simulink model "Vehicle_Control_CodeGen"  (R2024a)
settings: Solver=FixedStepAuto  StartTime=0.0  StopTime=10  RelTol=1e-3  EnableMultiTasking=on
undefined symbols (not defined in the file or in its folder): CAN, DiscIntNeverNeededParam, FD, Ion, Lithium
libraries: stmutilitieslib x28, simulink x21, stm32blockslib x10, canfdmsglib x6, dspstat3 x6, slpidlib x3, spsBatteryLib x2, spsControlledCurrentSourceLib x2, spsVoltageMeasurementLib x2, spspowerguiLib x2, stm32h7xxblockslib x2
(part 2 of 3)

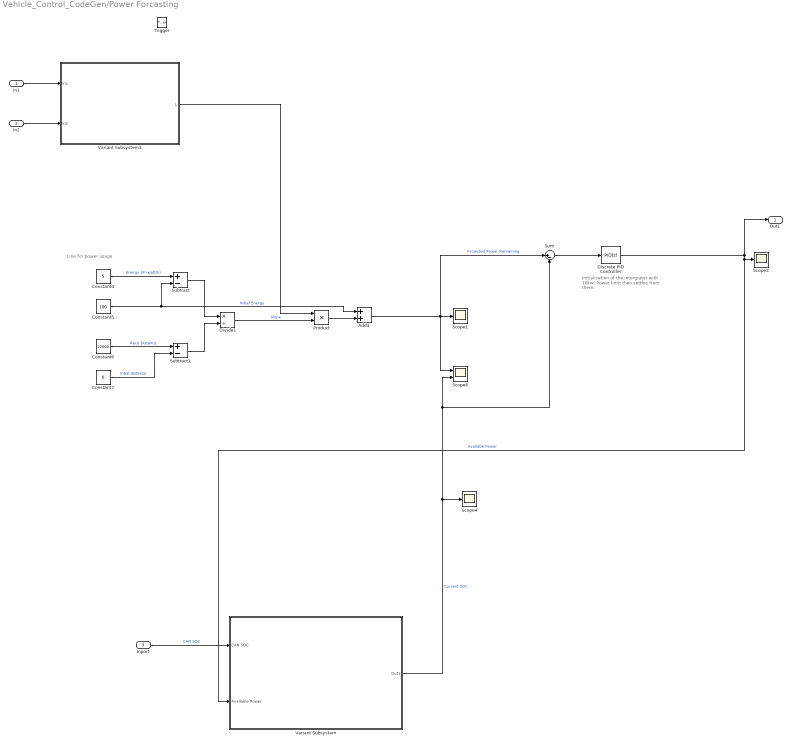
== system Vehicle_Control_CodeGen/Power Forcasting ==
  note: Line for power usage
  note: Initialisation of the intergrater with 10kw. Power limit then settles from there.
  In1 : Inport
  In2 : Inport  Port=2
  Inport : Inport  Port=3
  Trigger : TriggerPort  TriggerType=function-call  VariantControl=(inherit)
  Add3 : Sum
  Constant4 : Constant  Value=5
  Constant5 : Constant  Value=100
  Constant6 : Constant  Value=22000
  Constant7 : Constant  Value=0
  Discrete PID Controller : slpidlib/PID Controller  Controller=PID  Form=Parallel  TimeDomain=Discrete-time  UseExternalTs=off  SampleTime=-1  IntegratorMethod=Forward Euler  FilterMethod=Forward Euler  ControllerParametersSource=internal  P=-420  I=0.042  UseKiTs=off  D=21000  UseExternalDerivativeSource=off  N=0.01  UseFilter=on  TunerSelectOption=Transfer Function Based (PID Tuner App)  InitialConditionSource=internal  InitialConditionForIntegrator=10000  InitialConditionForFilter=0  DifferentiatorICPrevScaledInput=0  ExternalReset=none  TrackingMode=off  Kt=1  LimitOutput=off  SatLimitsSource=internal  UpperSaturationLimit=inf  LowerSaturationLimit=-inf  LinearizeAsGain=off  AntiWindupMode=none  Kb=1  LimitIntegrator=off  UpperIntegratorSaturationLimit=inf  LowerIntegratorSaturationLimit=-inf  POutMin=[]  POutMax=[]  IOutMin=[]  IOutMax=[]  DOutMin=[]  DOutMax=[]  NOutMin=[]  NOutMax=[]  SumOutMin=[]  SumOutMax=[]  SaturationOutMin=[]  SaturationOutMax=[]  PParamMin=[]  PParamMax=[]  IParamMin=[]  IParamMax=[]  DParamMin=[]  DParamMax=[]  NParamMin=[]  NParamMax=[]  KbParamMin=[]  KbParamMax=[]  KtParamMin=[]  KtParamMax=[]  KbOutMin=[]  KbOutMax=[]  KtOutMin=[]  KtOutMax=[]  IntegratorOutMin=[]  IntegratorOutMax=[]  FilterOutMin=[]  FilterOutMax=[]  SumI1OutMin=[]  SumI1OutMax=[]  SumI2OutMin=[]  SumI2OutMax=[]  SumI3OutMin=[]  SumI3OutMax=[]  SumI4OutMin=[]  SumI4OutMax=[]  SumDOutMin=[]  SumDOutMax=[]  DifferentiatorOutMin=[]  DifferentiatorOutMax=[]  FilterDiffOutCoefMin=[]  FilterDiffOutCoefMax=[]  ReciprocalOutMin=[]  ReciprocalOutMax=[]  SumDenOutMin=[]  SumDenOutMax=[]  SumNumOutMin=[]  SumNumOutMax=[]  DivideOutMin=[]  DivideOutMax=[]  UdiffTsProdOutMin=[]  UdiffTsProdOutMax=[]  NTsProdOutMin=[]  NTsProdOutMax=[]  UintegralTsProdOutMin=[]  UintegralTsProdOutMax=[]  UngainTsProdOutMin=[]  UngainTsProdOutMax=[]  ClampingZeroOutDataTypeStr=Inherit: Inherit via back propagation  ClampingZeroOutMin=[]  ClampingZeroOutMax=[]  FilterDenConstantOutDataTypeStr=Inherit: Inherit via back propagation  FilterDenConstantOutMin=[]  FilterDenConstantOutMax=[]  PCopyOutDataTypeStr=Inherit: Inherit via back propagation  PCopyOutMin=[]  PCopyOutMax=[]  NCopyOutDataTypeStr=Inherit: Inherit via back propagation  NCopyOutMin=[]  NCopyOutMax=[]  IntegratorContinuousStateAttributes=''  IntegratorStateMustResolveToSignalObject=off  IntegratorRTWStateStorageClass=Auto  FilterContinuousStateAttributes=''  FilterStateMustResolveToSignalObject=off  FilterRTWStateStorageClass=Auto  ParallelPVariant=InternalParameters  IdealPVariant=Disabled  IVariant=InternalParameters  DVariant=InternalParameters  IntegratorVariant=Discrete  SatVariant=Disabled  AWVariant=Passthrough  PCopyVariant=Disabled  TRVariant=Disabled  FdbkBlocksVariant=Forward  IdealPFdbkVariant=Disabled  SatFdbkVariant=Disabled  DerivativeFilterVariant=ForwardEulerFilter  NVariant=InternalParameters  NCopyVariant=Disabled  FilterICVariant=InternalICsFilter  IntegratorICVariant=InternalICs  ExternalResetVariant=Disabled  TRSumVariant=Passthrough  SumFdbkVariant=Disabled  SumVariant=Sum_PID  TsampFilterVariant=InternalTs  TsampNgainVariant=Passthrough  TsampIntegralVariant=Disabled_SignalSpec  ExternalSaturationOutDataTypeStr=Inherit: Same as second input  DerivativeSourceVariant=ErrorSignal
      settings: LibrarySourceBlock=simulink/Discrete/Discrete PID Controller
  Divide1 : Product  Inputs=*/
  Product : Product
  Scope1 : Scope
  Scope3 : Scope
  Scope4 : Scope
  Scope6 : Scope  NumInputPorts=2
  Subtract : Sum  Inputs=+-
  Subtract1 : Sum  Inputs=+-
  Sum : Sum  Inputs=|+-
  Variant Subsystem : Subsystem  Variant=on  VariantControlMode=sim codegen switching
  Variant Subsystem1 : Subsystem  Variant=on  VariantControlMode=sim codegen switching
  Out1 : Outport
  wires:
  In1/1 -> Variant Subsystem1/1(In1)
  In2/1 -> Variant Subsystem1/2(In2)
  Variant Subsystem/1(Out1) -> Scope4/1, Sum/2, Scope6/2  "Current SOC"
  Variant Subsystem1/1(1) -> Product/1
  Constant7/1 -> Subtract1/2  "Intial distance"
  Sum/1 -> Discrete PID Controller/1
  Divide1/1 -> Product/2  "Slope"
  Subtract1/1 -> Divide1/2
  Product/1 -> Add3/2
  Add3/1 -> Scope6/1, Sum/1, Scope1/1  "Projected Power Remaining"
  Constant4/1 -> Subtract/1  "Energy SF (watt/h)"
  Discrete PID Controller/1 -> Variant Subsystem/2(Available Power), Scope3/1, Out1/1  "Availabe Power"
  Constant5/1 -> Add3/1, Subtract/2  "Initial Energy"
  Subtract/1 -> Divide1/1
  Constant6/1 -> Subtract1/1  "Race Distance"
  Inport/1 -> Variant Subsystem/1(CAN SOC)  "CAN SOC"

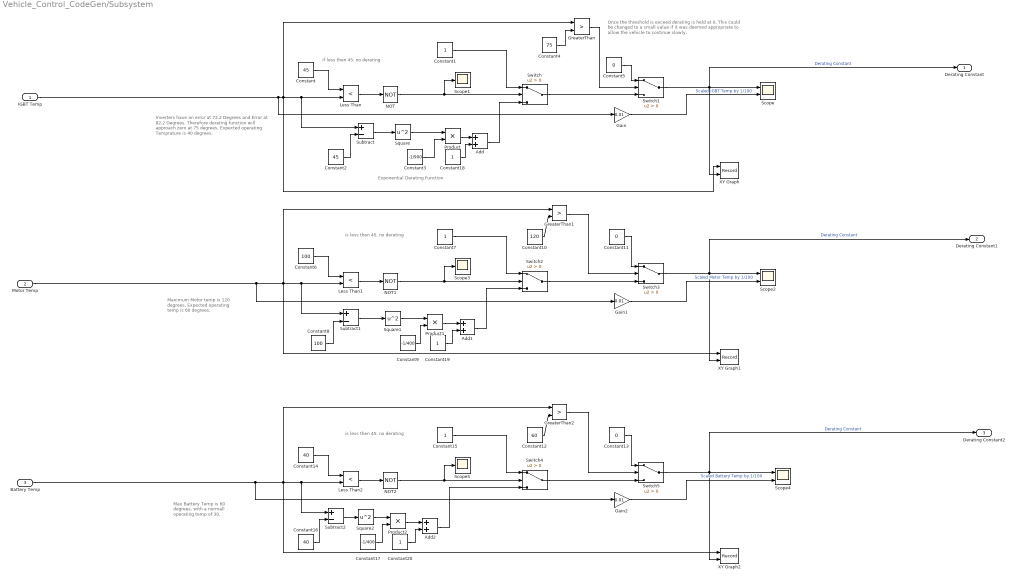
== system Vehicle_Control_CodeGen/Subsystem ==
  note: Once the threshold is exceed derating is held at 0, This could be changed to a small value if it was deemed appropriate to allow the vehicle to continue slowly.
  note: Exponential Derating Function
  note: if less then 45, no derating
  note: Max Battery Temp is 60 degrees, with a normall operating temp of 30.
  note: Maximum Motor temp is 120 degrees. Expected operating temp is 60 degrees.
  note: Inverters have an error at 72.2 Degrees and Error at 82.2 Degrees. Therefore derating function will approach zero at 75 degrees. Expected operating Temprature is 40 degrees.
  note: is less then 45, no derating
  note: is less then 45, no derating
  IGBT Temp : Inport
  Motor Temp : Inport  Port=2
  Battery Temp : Inport  Port=3
  Add : Sum
  Add1 : Sum
  Add2 : Sum
  Constant : Constant  Value=45
  Constant{1,7,15,18..20} (6 alike) : Constant
  Constant10 : Constant  Value=120
  Constant11 : Constant  Value=0
  Constant12 : Constant  Value=60
  Constant13 : Constant  Value=0
  Constant14 : Constant  Value=40
  Constant16 : Constant  Value=40
  Constant17 : Constant  Value=-1/400
  Constant2 : Constant  Value=45
  Constant3 : Constant  Value=-1/900
  Constant4 : Constant  Value=75
  Constant5 : Constant  Value=0
  Constant6 : Constant  Value=100
  Constant8 : Constant  Value=100
  Constant9 : Constant  Value=-1/400
  Gain : Gain  Gain=0.01
  Gain1 : Gain  Gain=0.01
  Gain2 : Gain  Gain=0.01
  GreaterThan : RelationalOperator  Operator=>  OutDataTypeStr=boolean  RndMeth=Simplest  InputSameDT=off
  GreaterThan1 : RelationalOperator  Operator=>  OutDataTypeStr=boolean  RndMeth=Simplest  InputSameDT=off
  GreaterThan2 : RelationalOperator  Operator=>  OutDataTypeStr=boolean  RndMeth=Simplest  InputSameDT=off
  Less Than : RelationalOperator  Operator=<  OutDataTypeStr=boolean  RndMeth=Simplest  InputSameDT=off
  Less Than1 : RelationalOperator  Operator=<  OutDataTypeStr=boolean  RndMeth=Simplest  InputSameDT=off
  Less Than2 : RelationalOperator  Operator=<  OutDataTypeStr=boolean  RndMeth=Simplest  InputSameDT=off
  NOT : Logic  Operator=NOT  IconShape=distinctive  AllPortsSameDT=off  OutDataTypeStr=boolean
  NOT1 : Logic  Operator=NOT  IconShape=distinctive  AllPortsSameDT=off  OutDataTypeStr=boolean
  NOT2 : Logic  Operator=NOT  IconShape=distinctive  AllPortsSameDT=off  OutDataTypeStr=boolean
  Product : Product
  Product1 : Product
  Product2 : Product
  Scope : Scope  NumInputPorts=2
  Scope1 : Scope
  Scope2 : Scope  NumInputPorts=2
  Scope3 : Scope
  Scope4 : Scope  NumInputPorts=2
  Scope5 : Scope
  Square : Math  Operator=square
  Square1 : Math  Operator=square
  Square2 : Math  Operator=square
  Subtract : Sum  Inputs=+-
  Subtract1 : Sum  Inputs=+-
  Subtract2 : Sum  Inputs=+-
  Switch{,1..5} (6 alike) : Switch  Criteria=u2 > Threshold  SaturateOnIntegerOverflow=off  InputSameDT=off
  XY Graph : Record  FileSettingsInternal="{\"entries\":[{\"content\":{\"excelSettings\":{\"content\":{},\"type\":\"Streamout.ExcelSettings\"}},\"type\":\"Streamout.FileSettingStorage\",\"uuid\":\"\"}],\"packageUris\":[\"http:\\/\\/schema.mathworks.com\\/mf0\\/streamout_blocks\\/R2020a\"],\"version\":\"1.0\"}"  Layout=[1 1]  SignalsInternal="{\"entries\":[{\"content\":{\"signals\":[{\"content\":{\"blockPath\":[],\"dimensions\":[1],\"domain\":\"\",\"lineColor\":\"#a2142f\",\"plots\":[ 1 ],\"port\":1,\"signalID\":1,\"signalName\":\"IGBT Temp\"},\"type\":\"RecordBlkView.Signal\",\"uuid\":\"\"},{\"content\":{\"blockPath\":[],\"dimensions\":[1],\"domain\":\"\",\"lineColor\":\"#139fff\",\"plots\":[ 1 ],\"port\":2,\"signalID\":2,\"signalName\":\"Derating Constant\"},\"type\":\"RecordBlkView.Signal\",\"uuid\":\"\"}]},\"type\":\"RecordBlkView.InputSignals\",\"uuid\":\"\"}],\"packageUris\":[\"http:\\/\\/schema.mathworks.com\\/mf0\\/streamout_blocks\\/R2020a\"],\"version\":\"1.0\"}"  VisualizationBindings="{\"xyplotplugin\":{\"info\":[{\"series\":[{\"bindingParametersList\":[{\"parameter\":\"X-Axis\",\"signalID\":1,\"signalName\":\"IGBT Temp\"},{\"parameter\":\"Y-Axis\",\"signalID\":2,\"signalName\":\"Derating Constant\"}],\"seriesID\":0}],\"subplotID\":1}]}}"  CompatibilityTag=XY
  XY Graph1 : Record  FileSettingsInternal="{\"entries\":[{\"content\":{\"excelSettings\":{\"content\":{},\"type\":\"Streamout.ExcelSettings\"}},\"type\":\"Streamout.FileSettingStorage\",\"uuid\":\"\"}],\"packageUris\":[\"http:\\/\\/schema.mathworks.com\\/mf0\\/streamout_blocks\\/R2020a\"],\"version\":\"1.0\"}"  Layout=[1 1]  SignalsInternal="{\"entries\":[{\"content\":{\"signals\":[{\"content\":{\"blockPath\":[],\"dimensions\":[1],\"domain\":\"\",\"lineColor\":\"#a2142f\",\"plots\":[ 1 ],\"port\":1,\"signalID\":1,\"signalName\":\"Motor Temp\"},\"type\":\"RecordBlkView.Signal\",\"uuid\":\"\"},{\"content\":{\"blockPath\":[],\"dimensions\":[1],\"domain\":\"\",\"lineColor\":\"#139fff\",\"plots\":[ 1 ],\"port\":2,\"signalID\":2,\"signalName\":\"Derating Constant\"},\"type\":\"RecordBlkView.Signal\",\"uuid\":\"\"}]},\"type\":\"RecordBlkView.InputSignals\",\"uuid\":\"\"}],\"packageUris\":[\"http:\\/\\/schema.mathworks.com\\/mf0\\/streamout_blocks\\/R2020a\"],\"version\":\"1.0\"}"  VisualizationBindings="{\"xyplotplugin\":{\"info\":[{\"series\":[{\"bindingParametersList\":[{\"parameter\":\"X-Axis\",\"signalID\":1,\"signalName\":\"Motor Temp\"},{\"parameter\":\"Y-Axis\",\"signalID\":2,\"signalName\":\"Derating Constant\"}],\"seriesID\":0}],\"subplotID\":1}]}}"  CompatibilityTag=XY
  XY Graph2 : Record  FileSettingsInternal="{\"entries\":[{\"content\":{\"excelSettings\":{\"content\":{},\"type\":\"Streamout.ExcelSettings\"}},\"type\":\"Streamout.FileSettingStorage\",\"uuid\":\"\"}],\"packageUris\":[\"http:\\/\\/schema.mathworks.com\\/mf0\\/streamout_blocks\\/R2020a\"],\"version\":\"1.0\"}"  Layout=[1 1]  SignalsInternal="{\"entries\":[{\"content\":{\"signals\":[{\"content\":{\"blockPath\":[],\"dimensions\":[1],\"domain\":\"\",\"lineColor\":\"#a2142f\",\"plots\":[ 1 ],\"port\":1,\"signalID\":1,\"signalName\":\"Battery Temp\"},\"type\":\"RecordBlkView.Signal\",\"uuid\":\"\"},{\"content\":{\"blockPath\":[],\"dimensions\":[1],\"domain\":\"\",\"lineColor\":\"#139fff\",\"plots\":[ 1 ],\"port\":2,\"signalID\":2,\"signalName\":\"Derating Constant\"},\"type\":\"RecordBlkView.Signal\",\"uuid\":\"\"}]},\"type\":\"RecordBlkView.InputSignals\",\"uuid\":\"\"}],\"packageUris\":[\"http:\\/\\/schema.mathworks.com\\/mf0\\/streamout_blocks\\/R2020a\"],\"version\":\"1.0\"}"  VisualizationBindings="{\"xyplotplugin\":{\"info\":[{\"series\":[{\"bindingParametersList\":[{\"parameter\":\"X-Axis\",\"signalID\":1,\"signalName\":\"Battery Temp\"},{\"parameter\":\"Y-Axis\",\"signalID\":2,\"signalName\":\"Derating Constant\"}],\"seriesID\":0}],\"subplotID\":1}]}}"  CompatibilityTag=XY
  Derating Constant : Outport
  Derating Constant1 : Outport  Port=2
  Derating Constant2 : Outport  Port=3
  wires:
  Add/1 -> Switch/3
  Less Than2/1 -> NOT2/1
  Motor Temp/1 -> XY Graph1/1, GreaterThan1/1, Subtract1/1, Less Than1/2, Gain1/1
  NOT2/1 -> Scope5/1, Switch4/2
  Constant7/1 -> Switch2/1
  Switch1/1 -> Derating Constant/1, Scope/1, XY Graph/2  "Derating Constant"
  Gain1/1 -> Scope2/2  "Scaled Motor Temp by 1/100"
  NOT1/1 -> Scope3/1, Switch2/2
  GreaterThan/1 -> Switch1/2
  Constant18/1 -> Add/2
  Constant16/1 -> Subtract2/2
  Subtract1/1 -> Square1/1
  Constant1/1 -> Switch/1
  Battery Temp/1 -> XY Graph2/1, GreaterThan2/1, Subtract2/1, Less Than2/2, Gain2/1
  Subtract2/1 -> Square2/1
  Constant5/1 -> Switch1/1
  Switch/1 -> Switch1/3
  Less Than/1 -> NOT/1
  Product1/1 -> Add1/1
  Constant2/1 -> Subtract/2
  Constant6/1 -> Less Than1/1
  Subtract/1 -> Square/1
  Gain2/1 -> Scope4/2  "Scaled Battery Temp by 1/100"
  Add1/1 -> Switch2/3
  Add2/1 -> Switch4/3
  Constant19/1 -> Add1/2
  Constant8/1 -> Subtract1/2
  Square/1 -> Product/1
  Constant9/1 -> Product1/2
  Constant4/1 -> GreaterThan/2
  IGBT Temp/1 -> Gain/1, XY Graph/1, GreaterThan/1, Subtract/1, Less Than/2
  Constant10/1 -> GreaterThan1/2
  Gain/1 -> Scope/2  "Scaled IGBT Temp by 1/100"
  Switch2/1 -> Switch3/3
  Switch3/1 -> Derating Constant1/1, Scope2/1, XY Graph1/2  "Derating Constant"
  Constant3/1 -> Product/2
  Constant14/1 -> Less Than2/1
  Constant20/1 -> Add2/2
  Switch4/1 -> Switch5/3
  Square1/1 -> Product1/1
  Less Than1/1 -> NOT1/1
  Constant11/1 -> Switch3/1
  Constant12/1 -> GreaterThan2/2
  Square2/1 -> Product2/1
  GreaterThan1/1 -> Switch3/2
  Switch5/1 -> Derating Constant2/1, Scope4/1, XY Graph2/2  "Derating Constant"
  Constant13/1 -> Switch5/1
  Product/1 -> Add/1
  Constant/1 -> Less Than/1
  Constant15/1 -> Switch4/1
  NOT/1 -> Scope1/1, Switch/2
  Product2/1 -> Add2/1
  Constant17/1 -> Product2/2
  GreaterThan2/1 -> Switch5/2

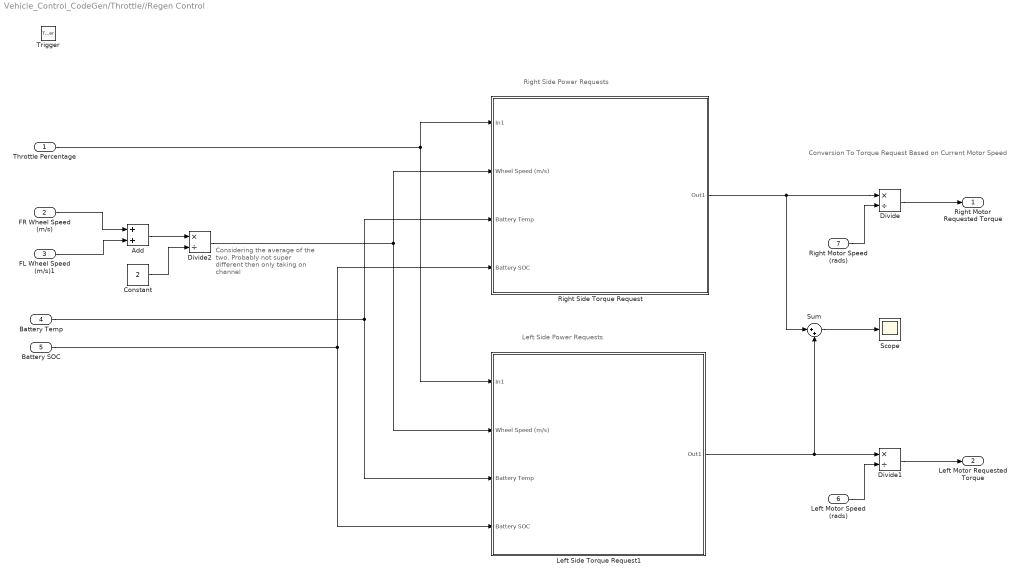
== system Vehicle_Control_CodeGen/Throttle//Regen Control ==
  note: Conversion To Torque Request Based on Current Motor Speed
  note: Right Side Power Requests
  note: Considering the average of the two. Probably not super different then only taking on channel
  note: Left Side Power Requests
  Throttle Percentage : Inport
  FR Wheel Speed (m/s) : Inport  Port=2
  FL Wheel Speed (m/s)1 : Inport  Port=3
  Battery Temp : Inport  Port=4
  Battery SOC : Inport  Port=5
  Left Motor Speed (rads) : Inport  Port=6
  Right Motor Speed (rads) : Inport  Port=7
  Trigger : TriggerPort  TriggerType=function-call  VariantControl=(inherit)
  Add : Sum
  Constant : Constant  Value=2
  Divide : Product  Inputs=*/
  Divide1 : Product  Inputs=*/
  Divide2 : Product  Inputs=*/
  Left Side Torque Request1 : Subsystem
  Right Side Torque Request : Subsystem
  Scope : Scope
  Sum : Sum  Inputs=|++
  Right Motor Requested Torque : Outport
  Left Motor Requested Torque : Outport  Port=2
  wires:
  Right Side Torque Request/1(Out1) -> Sum/1, Divide/1
  Divide/1 -> Right Motor Requested Torque/1
  Left Motor Speed (rads)/1 -> Divide1/2
  Sum/1 -> Scope/1
  Left Side Torque Request1/1(Out1) -> Divide1/1, Sum/2
  Divide1/1 -> Left Motor Requested Torque/1
  Throttle Percentage/1 -> Left Side Torque Request1/1(In1), Right Side Torque Request/1(In1)
  Right Motor Speed (rads)/1 -> Divide/2
  Divide2/1 -> Right Side Torque Request/2(Wheel Speed (m/s)), Left Side Torque Request1/2(Wheel Speed (m/s))
  Battery Temp/1 -> Right Side Torque Request/3(Battery Temp), Left Side Torque Request1/3(Battery Temp)
  Battery SOC/1 -> Right Side Torque Request/4(Battery SOC), Left Side Torque Request1/4(Battery SOC)
  FR Wheel Speed (m/s)/1 -> Add/1
  FL Wheel Speed (m/s)1/1 -> Add/2
  Add/1 -> Divide2/1
  Constant/1 -> Divide2/2

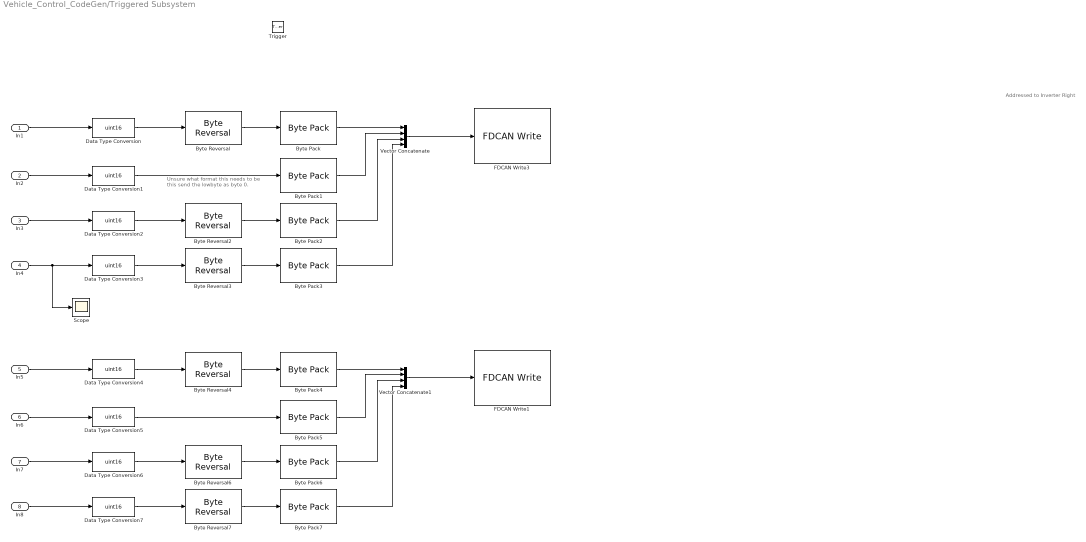
== system Vehicle_Control_CodeGen/Triggered Subsystem ==
  note: Unsure what format this needs to be this send the lowbyte as byte 0.
  note: Addressed to Inverter Right
  In1 : Inport
  In2 : Inport  Port=2
  In3 : Inport  Port=3
  In4 : Inport  Port=4
  In5 : Inport  Port=5
  In6 : Inport  Port=6
  In7 : Inport  Port=7
  In8 : Inport  Port=8
  Trigger : TriggerPort  TriggerType=function-call  VariantControl=(inherit)
  Byte Pack{,1..7} (8 alike) : stmutilitieslib/Byte Pack  datatypes={'uint16'}  byteAlign=1  blockPlatform=stm32f4discovery
  Byte Reversal{,2..4,6..7} (6 alike) : stmutilitieslib/Byte Reversal  numInp=1  blockPlatform=stm32f4discovery
  Data Type Conversion{,1..7} (8 alike) : DataTypeConversion  OutDataTypeStr=uint16  SaturateOnIntegerOverflow=off  RndMeth=Floor
  FDCAN Write1 : stm32blockslib/FDCAN Write  FDCANModule=FDCAN2  BlockMode=Transmit  OperationReadMode=Data  OperationWriteMode=Data  ReadSource=FIFO 0  BufferNumber=0  OutputTypeReadMode=Unpacked  DataFormatWriteMode=Raw data  CANFrameType=CAN  IdentifierTypeVia=Dialog  IdentifierType=Standard (11-bit identifier)  IdentifierVia=Dialog  Identifier=9  DataLengthVia=Dialog  DataLength=8  OutputIdType=off  IsBitRateSwitchingEnabled=off  TransmitRemoteFrame=off  OutputFrameType=off  OutputBRS=off  OutputRemoteFrame=off  OutputTxFifoLevel=off  OutputRxFifoLevel=off  OutputStatus=off  Timeout=1  SampleTime=-1
      settings: LibrarySourceBlock=stm32l5xxblockslib/FDCAN Write
  FDCAN Write3 : stm32blockslib/FDCAN Write  FDCANModule=FDCAN2  BlockMode=Transmit  OperationReadMode=Data  OperationWriteMode=Data  ReadSource=FIFO 0  BufferNumber=0  OutputTypeReadMode=Unpacked  DataFormatWriteMode=Raw data  CANFrameType=CAN  IdentifierTypeVia=Dialog  IdentifierType=Standard (11-bit identifier)  IdentifierVia=Dialog  Identifier=8  DataLengthVia=Dialog  DataLength=8  OutputIdType=off  IsBitRateSwitchingEnabled=off  TransmitRemoteFrame=off  OutputFrameType=off  OutputBRS=off  OutputRemoteFrame=off  OutputTxFifoLevel=off  OutputRxFifoLevel=off  OutputStatus=off  Timeout=1  SampleTime=-1
      settings: LibrarySourceBlock=stm32l5xxblockslib/FDCAN Write
  Scope : Scope
  Vector Concatenate : Concatenate  NumInputs=4
  Vector Concatenate1 : Concatenate  NumInputs=4
  wires:
  Byte Reversal/1 -> Byte Pack/1
  Byte Pack/1 -> Vector Concatenate/1
  Data Type Conversion/1 -> Byte Reversal/1
  In1/1 -> Data Type Conversion/1
  Byte Pack1/1 -> Vector Concatenate/2
  Byte Pack2/1 -> Vector Concatenate/3
  Byte Reversal2/1 -> Byte Pack2/1
  Data Type Conversion2/1 -> Byte Reversal2/1
  Byte Pack3/1 -> Vector Concatenate/4
  Byte Reversal3/1 -> Byte Pack3/1
  Data Type Conversion3/1 -> Byte Reversal3/1
  In3/1 -> Data Type Conversion2/1
  In4/1 -> Scope/1, Data Type Conversion3/1
  Vector Concatenate/1 -> FDCAN Write3/1
  Byte Pack6/1 -> Vector Concatenate1/3
  Byte Reversal7/1 -> Byte Pack7/1
  Vector Concatenate1/1 -> FDCAN Write1/1
  Byte Pack5/1 -> Vector Concatenate1/2
  Byte Pack7/1 -> Vector Concatenate1/4
  Byte Pack4/1 -> Vector Concatenate1/1
  Data Type Conversion7/1 -> Byte Reversal7/1
  Data Type Conversion4/1 -> Byte Reversal4/1
  Data Type Conversion5/1 -> Byte Pack5/1
  Byte Reversal6/1 -> Byte Pack6/1
  Data Type Conversion6/1 -> Byte Reversal6/1
  Byte Reversal4/1 -> Byte Pack4/1
  In8/1 -> Data Type Conversion7/1
  In7/1 -> Data Type Conversion6/1
  In6/1 -> Data Type Conversion5/1
  In5/1 -> Data Type Conversion4/1
  Data Type Conversion1/1 -> Byte Pack1/1
  In2/1 -> Data Type Conversion1/1

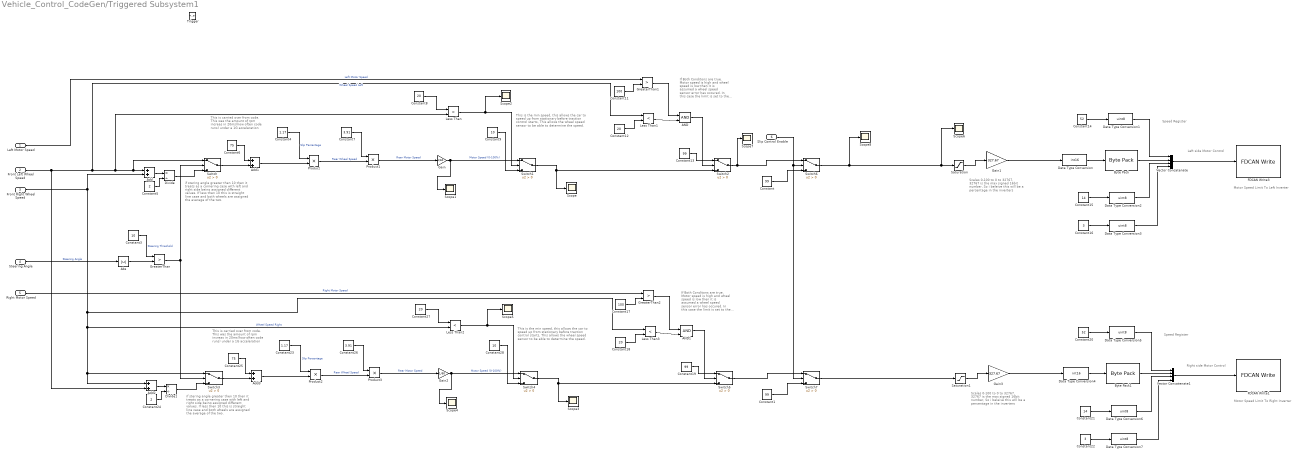
== system Vehicle_Control_CodeGen/Triggered Subsystem1 ==
  note: Scales 0-100 to 0 to 32767, 32767 is the max signed 16bit number, So i beleive this will be a percentage in the inverters
  note: Left side Motor Control
  note: If Both Conditons are true. Motor speed is high and wheel speed is low then it is assumed a wheel speed sensor error has occured. In this case the limit is set to the maximum.
  note: Speed Register
  note: Speed Register
  note: if stering angle greater then 10 then it treats as a cornering case with left and right side being assigned different values. If less then 10 this is straight line case and both wheels are assigned the average of the two.
  note: This is carried over from code. This was the amount of rpm increas in 20ms(how often code runs) under a 1G acceleration
  note: This is the min speed, this allows the car to speed up from stationary before traction control starts, This allows the wheel speed sensor to be able to determine the speed.
  note: if stering angle greater then 10 then it treats as a cornering case with left and right side being assigned different values. If less then 10 this is straight line case and both wheels are assigned the average of the two.
  note: This is the min speed, this allows the car to speed up from stationary before traction control starts, This allows the wheel speed sensor to be able to determine the speed.
  note: If Both Conditons are true. Motor speed is high and wheel speed is low then it is assumed a wheel speed sensor error has occured. In this case the limit is set to the maximum.
  note: Right side Motor Control
  note: Scales 0-100 to 0 to 32767, 32767 is the max signed 16bit number, So i beleive this will be a percentage in the inverters
  note: This is carried over from code. This was the amount of rpm increas in 20ms(how often code runs) under a 1G acceleration
  note: Motor Speed Limit To Right Inverter
  note: Motor Speed Limit To Left Inverter
  Left Motor Speed : Inport
  Front Left Wheel Speed : Inport  Port=2
  Front Right Wheel Speed : Inport  Port=3
  Steering Angle : Inport  Port=4
  Right Motor Speed : Inport  Port=5
  Slip Control Enable : Inport  Port=6
  Trigger : TriggerPort  TriggerType=function-call  VariantControl=(inherit)
  AND : Logic  IconShape=distinctive  AllPortsSameDT=off  OutDataTypeStr=boolean
  AND1 : Logic  IconShape=distinctive  AllPortsSameDT=off  OutDataTypeStr=boolean
  Abs : Abs  SaturateOnIntegerOverflow=off
  Add{,1..3} (4 alike) : Sum
  Byte Pack : stmutilitieslib/Byte Pack  datatypes={'int16'}  byteAlign=1  blockPlatform=stm32f4discovery
  Byte Pack1 : stmutilitieslib/Byte Pack  datatypes={'int16'}  byteAlign=1  blockPlatform=stm32f4discovery
  Constant{,1,13,19} (4 alike) : Constant  Value=99
  Constant11 : Constant  Value=100
  Constant{8,12,18,27} (4 alike) : Constant  Value=20
  Constant14 : Constant  Value=52
  Constant15 : Constant  Value=14
  Constant16 : Constant  Value=3
  Constant17 : Constant  Value=100
  Constant20 : Constant  Value=52
  Constant21 : Constant  Value=14
  Constant22 : Constant  Value=3
  Constant23 : Constant  Value=1.17
  Constant24 : Constant  Value=2
  Constant25 : Constant  Value=75
  Constant26 : Constant  Value=3.91
  Constant28 : Constant  Value=10
  Constant3 : Constant  Value=10
  Constant4 : Constant  Value=1.17
  Constant5 : Constant  Value=2
  Constant6 : Constant  Value=75
  Constant7 : Constant  Value=3.91
  Constant9 : Constant  Value=10
  Data Type Conversion : DataTypeConversion  OutDataTypeStr=int16  SaturateOnIntegerOverflow=off  RndMeth=Floor
  Data Type Conversion{1..3,5..7} (6 alike) : DataTypeConversion  OutDataTypeStr=uint8  SaturateOnIntegerOverflow=off  RndMeth=Floor
  Data Type Conversion4 : DataTypeConversion  OutDataTypeStr=int16  SaturateOnIntegerOverflow=off  RndMeth=Floor
  Divide : Product  Inputs=*/
  Divide1 : Product  Inputs=*/
  FDCAN Write1 : stm32blockslib/FDCAN Write  FDCANModule=FDCAN2  BlockMode=Transmit  OperationReadMode=Data  OperationWriteMode=Data  ReadSource=FIFO 0  BufferNumber=0  OutputTypeReadMode=Unpacked  DataFormatWriteMode=Raw data  CANFrameType=CAN  IdentifierTypeVia=Dialog  IdentifierType=Standard (11-bit identifier)  IdentifierVia=Dialog  Identifier=529  DataLengthVia=Dialog  DataLength=3  OutputIdType=off  IsBitRateSwitchingEnabled=off  TransmitRemoteFrame=off  OutputFrameType=off  OutputBRS=off  OutputRemoteFrame=off  OutputTxFifoLevel=off  OutputRxFifoLevel=off  OutputStatus=off  Timeout=1  SampleTime=-1
      settings: LibrarySourceBlock=stm32l5xxblockslib/FDCAN Write
  FDCAN Write3 : stm32blockslib/FDCAN Write  FDCANModule=FDCAN2  BlockMode=Transmit  OperationReadMode=Data  OperationWriteMode=Data  ReadSource=FIFO 0  BufferNumber=0  OutputTypeReadMode=Unpacked  DataFormatWriteMode=Raw data  CANFrameType=CAN  IdentifierTypeVia=Dialog  IdentifierType=Standard (11-bit identifier)  IdentifierVia=Dialog  Identifier=528  DataLengthVia=Dialog  DataLength=3  OutputIdType=off  IsBitRateSwitchingEnabled=off  TransmitRemoteFrame=off  OutputFrameType=off  OutputBRS=off  OutputRemoteFrame=off  OutputTxFifoLevel=off  OutputRxFifoLevel=off  OutputStatus=off  Timeout=1  SampleTime=-1
      settings: LibrarySourceBlock=stm32l5xxblockslib/FDCAN Write
  Gain : Gain  Gain=1/60
  Gain1 : Gain  Gain=327.67
  Gain2 : Gain  Gain=1/60
  Gain3 : Gain  Gain=327.67
  GreaterThan : RelationalOperator  Operator=>  OutDataTypeStr=boolean  RndMeth=Simplest  InputSameDT=off
  GreaterThan1 : RelationalOperator  Operator=>  OutDataTypeStr=boolean  RndMeth=Simplest  InputSameDT=off
  GreaterThan2 : RelationalOperator  Operator=>  OutDataTypeStr=boolean  RndMeth=Simplest  InputSameDT=off
  Less Than{,1..3} (4 alike) : RelationalOperator  Operator=<  OutDataTypeStr=boolean  RndMeth=Simplest  InputSameDT=off
  Product{,1..3} (4 alike) : Product
  Saturation : Saturate  UpperLimit=99  LowerLimit=0
  Saturation1 : Saturate  UpperLimit=99  LowerLimit=0
  Scope{,1..8} (9 alike) : Scope
  Switch{,1..7} (8 alike) : Switch  Criteria=u2 > Threshold  SaturateOnIntegerOverflow=off  InputSameDT=off
  Vector Concatenate : Concatenate  NumInputs=4
  Vector Concatenate1 : Concatenate  NumInputs=4
  wires:
  Product3/1 -> Gain2/1  "Rear Motor Speed"
  Constant18/1 -> Less Than3/2
  Constant20/1 -> Data Type Conversion5/1
  Front Right Wheel Speed/1 -> Add/2, Less Than2/2, Add2/1, Switch3/1, Less Than3/1  "Wheel Speed Right"
  Byte Pack/1 -> Vector Concatenate/2
  Constant14/1 -> Data Type Conversion1/1
  Constant25/1 -> Add3/1
  GreaterThan/1 -> Switch3/2, Switch/2
  Constant26/1 -> Product3/1
  Front Left Wheel Speed/1 -> Add2/2, Less Than1/1, Less Than/2, Switch/1, Add/1  "Wheel Speed Left"
  Gain2/1 -> Switch4/1, Scope4/1  "Motor Speed (0-100%)"
  Product2/1 -> Product3/2  "Rear Wheel Speed"
  Constant19/1 -> Switch5/1
  Constant24/1 -> Divide1/2
  Product/1 -> Product1/2  "Rear Wheel Speed"
  Constant23/1 -> Product2/1  "Slip Percentage"
  Data Type Conversion7/1 -> Vector Concatenate1/4
  Add1/1 -> Product/2
  Constant21/1 -> Data Type Conversion6/1
  Less Than3/1 -> AND1/2
  Switch4/1 -> Switch5/3, Scope3/1
  Add2/1 -> Divide1/1
  Constant12/1 -> Less Than1/2
  AND1/1 -> Switch5/2
  Byte Pack1/1 -> Vector Concatenate1/2
  Switch7/1 -> Saturation1/1
  Data Type Conversion4/1 -> Byte Pack1/1
  Constant8/1 -> Less Than/1
  Constant16/1 -> Data Type Conversion3/1
  Constant15/1 -> Data Type Conversion2/1
  Data Type Conversion1/1 -> Vector Concatenate/1
  Data Type Conversion/1 -> Byte Pack/1
  Less Than1/1 -> AND/2
  Switch3/1 -> Add3/2
  Constant7/1 -> Product1/1
  Add3/1 -> Product2/2
  GreaterThan1/1 -> AND/1
  Abs/1 -> GreaterThan/2
  Left Motor Speed/1 -> GreaterThan1/1  "Left Motor Speed"
  Constant11/1 -> GreaterThan1/2
  Switch6/1 -> Scope8/1, Scope6/1, Saturation/1
  Product1/1 -> Gain/1  "Rear Motor Speed"
  Divide/1 -> Switch/3
  Switch/1 -> Add1/2
  Add/1 -> Divide/1
  Switch1/1 -> Switch2/3, Scope/1
  Gain1/1 -> Data Type Conversion/1
  Constant9/1 -> Switch1/3
  Constant3/1 -> GreaterThan/1  "Steering Threshold"
  Constant5/1 -> Divide/2
  Data Type Conversion3/1 -> Vector Concatenate/4
  Gain/1 -> Switch1/1, Scope1/1  "Motor Speed (0-100%)"
  Constant6/1 -> Add1/1
  Constant28/1 -> Switch4/3
  Saturation/1 -> Gain1/1
  Less Than2/1 -> Switch4/2, Scope5/1
  Less Than/1 -> Switch1/2, Scope2/1
  Constant22/1 -> Data Type Conversion7/1
  Divide1/1 -> Switch3/3
  Constant4/1 -> Product/1  "Slip Percentage"
  Steering Angle/1 -> Abs/1  "Steering Angle"
  Constant17/1 -> GreaterThan2/2
  Saturation1/1 -> Gain3/1
  Data Type Conversion5/1 -> Vector Concatenate1/1
  Constant13/1 -> Switch2/1
  Constant27/1 -> Less Than2/1
  Gain3/1 -> Data Type Conversion4/1
  Right Motor Speed/1 -> GreaterThan2/1  "Right Motor Speed"
  AND/1 -> Switch2/2
  Data Type Conversion2/1 -> Vector Concatenate/3
  Data Type Conversion6/1 -> Vector Concatenate1/3
  GreaterThan2/1 -> AND1/1
  Vector Concatenate/1 -> FDCAN Write3/1
  Vector Concatenate1/1 -> FDCAN Write1/1
  Switch2/1 -> Scope7/1, Switch6/1
  Constant/1 -> Switch6/3
  Slip Control Enable/1 -> Switch6/2, Switch7/2
  Constant1/1 -> Switch7/3
  Switch5/1 -> Switch7/1

== system Vehicle_Control_CodeGen/Variant Subsystem ==
  note: 1) Add Subsystem or Model blocks as valid variant choices.
      | 2) You cannot connect blocks at this level. At simulation, connectivity is automatically
      | determined, based on the active variant and port name matching.
  In1 : Inport
  CAN Forwarding : Subsystem  VariantControl=(codegen)
  Simulation of Throttle Pedal : Subsystem  VariantControl=(sim)
  Out1 : Outport

== system Vehicle_Control_CodeGen/Variant Subsystem1 ==
  note: 1) Add Subsystem or Model blocks as valid variant choices.
      | 2) You cannot connect blocks at this level. At simulation, connectivity is automatically
      | determined, based on the active variant and port name matching.
  Can Sig : Inport
  Requested Current : Inport  Port=2
  Battery Model1 : Subsystem  VariantControl=(sim)
  CAN Forwarding : Subsystem  VariantControl=(codegen)
  Batt Out : Outport
  Scope : Outport  Port=2

== system Vehicle_Control_CodeGen/10 HZ Send1/Enabled Subsystem ==
  note: The corrsosponding frequency which a requested message ID should be sent back at.
  note: A look up table of CAN ID's which are used to request cyclic transmission of data from the inverters
  note: Byte 0 tells the inverters you are setting up cyclic messaging.
  note: Addressed to Inverter LEFT
  note: Counter Selects which ID to send
  note: Addressed to Inverter Right
  Enable : EnablePort
  Constant4 : Constant  Value=61
  Counter Limited : simulink/Sources/Counter Limited  uplimit=5  tsamp=-1
  Counter Limited1 : simulink/Sources/Counter Limited  uplimit=5  tsamp=-1
  Data Type Conversion1 : DataTypeConversion  OutDataTypeStr=double  SaturateOnIntegerOverflow=off  RndMeth=Floor
  Data Type Conversion16 : DataTypeConversion  OutDataTypeStr=double  SaturateOnIntegerOverflow=off  RndMeth=Floor
  Data Type Conversion2 : DataTypeConversion  OutDataTypeStr=uint8  SaturateOnIntegerOverflow=off  RndMeth=Floor
  Data Type Conversion3 : DataTypeConversion  OutDataTypeStr=uint8  SaturateOnIntegerOverflow=off  RndMeth=Floor
  Data Type Conversion4 : DataTypeConversion  OutDataTypeStr=uint8  SaturateOnIntegerOverflow=off  RndMeth=Floor
  Direct Lookup Table (n-D) : LookupNDDirect  NumberOfTableDimensions=1  Table=[235 74 168 73 95 138]
  Direct Lookup Table (n-D)1 : LookupNDDirect  NumberOfTableDimensions=1  Table=[235 74 168 73 95 138]
  FDCAN Write2 : stm32blockslib/FDCAN Write  FDCANModule=FDCAN2  BlockMode=Transmit  OperationReadMode=Data  OperationWriteMode=Data  ReadSource=FIFO 0  BufferNumber=0  OutputTypeReadMode=Unpacked  DataFormatWriteMode=Raw data  CANFrameType=CAN  IdentifierTypeVia=Dialog  IdentifierType=Standard (11-bit identifier)  IdentifierVia=Dialog  Identifier=529  DataLengthVia=Dialog  DataLength=3  OutputIdType=off  IsBitRateSwitchingEnabled=off  TransmitRemoteFrame=off  OutputFrameType=off  OutputBRS=off  OutputRemoteFrame=off  OutputTxFifoLevel=off  OutputRxFifoLevel=off  OutputStatus=off  Timeout=1  SampleTime=-1
      settings: LibrarySourceBlock=stm32l5xxblockslib/FDCAN Write
  FDCAN Write3 : stm32blockslib/FDCAN Write  FDCANModule=FDCAN2  BlockMode=Transmit  OperationReadMode=Data  OperationWriteMode=Data  ReadSource=FIFO 0  BufferNumber=0  OutputTypeReadMode=Unpacked  DataFormatWriteMode=Raw data  CANFrameType=CAN  IdentifierTypeVia=Dialog  IdentifierType=Standard (11-bit identifier)  IdentifierVia=Dialog  Identifier=528  DataLengthVia=Dialog  DataLength=3  OutputIdType=off  IsBitRateSwitchingEnabled=off  TransmitRemoteFrame=off  OutputFrameType=off  OutputBRS=off  OutputRemoteFrame=off  OutputTxFifoLevel=off  OutputRxFifoLevel=off  OutputStatus=off  Timeout=1  SampleTime=-1
      settings: LibrarySourceBlock=stm32l5xxblockslib/FDCAN Write
  Scope2 : Scope
  Scope3 : Scope
  Vector Concatenate : Concatenate  NumInputs=3
  wires:
  Direct Lookup Table (n-D)1/1 -> Data Type Conversion4/1, Scope3/1
  Data Type Conversion1/1 -> Direct Lookup Table (n-D)1/1
  Data Type Conversion16/1 -> Direct Lookup Table (n-D)/1
  Direct Lookup Table (n-D)/1 -> Data Type Conversion2/1, Scope2/1
  Counter Limited1/1 -> Data Type Conversion1/1
  Counter Limited/1 -> Data Type Conversion16/1
  Vector Concatenate/1 -> FDCAN Write2/1, FDCAN Write3/1
  Data Type Conversion3/1 -> Vector Concatenate/1
  Data Type Conversion4/1 -> Vector Concatenate/3
  Data Type Conversion2/1 -> Vector Concatenate/2
  Constant4/1 -> Data Type Conversion3/1

== system Vehicle_Control_CodeGen/Function-Call Subsystem/If Action Subsystem1 ==
  In1 : Inport
  Action Port : ActionPort  ActionPortLabel=case [ 138 ]:
  Out1 : Outport
  wires:
  In1/1 -> Out1/1

== system Vehicle_Control_CodeGen/Function-Call Subsystem/If Action Subsystem10 ==
  In1 : Inport
  Action Port : ActionPort  ActionPortLabel=case [ 168 ]:
  Out1 : Outport
  wires:
  In1/1 -> Out1/1

== system Vehicle_Control_CodeGen/Function-Call Subsystem/If Action Subsystem11 ==
  In1 : Inport
  Action Port : ActionPort  ActionPortLabel=case [ 74 ]:
  Out1 : Outport
  wires:
  In1/1 -> Out1/1

== system Vehicle_Control_CodeGen/Function-Call Subsystem/If Action Subsystem12 ==
  In1 : Inport
  Action Port : ActionPort  ActionPortLabel=case [ 235 ]:
  Out1 : Outport
  wires:
  In1/1 -> Out1/1

== system Vehicle_Control_CodeGen/Function-Call Subsystem/If Action Subsystem2 ==
  In1 : Inport
  Action Port : ActionPort  ActionPortLabel=case [ 95 ]:
  Out1 : Outport
  wires:
  In1/1 -> Out1/1

== system Vehicle_Control_CodeGen/Function-Call Subsystem/If Action Subsystem3 ==
  In1 : Inport
  Action Port : ActionPort  ActionPortLabel=case [ 73 ]:
  Out1 : Outport
  wires:
  In1/1 -> Out1/1

== system Vehicle_Control_CodeGen/Function-Call Subsystem/If Action Subsystem4 ==
  In1 : Inport
  Action Port : ActionPort  ActionPortLabel=case [ 168 ]:
  Out1 : Outport
  wires:
  In1/1 -> Out1/1

== system Vehicle_Control_CodeGen/Function-Call Subsystem/If Action Subsystem5 ==
  In1 : Inport
  Action Port : ActionPort  ActionPortLabel=case [ 74 ]:
  Out1 : Outport
  wires:
  In1/1 -> Out1/1

== system Vehicle_Control_CodeGen/Function-Call Subsystem/If Action Subsystem6 ==
  In1 : Inport
  Action Port : ActionPort  ActionPortLabel=case [ 235 ]:
  Out1 : Outport
  wires:
  In1/1 -> Out1/1

== system Vehicle_Control_CodeGen/Function-Call Subsystem/If Action Subsystem7 ==
  In1 : Inport
  Action Port : ActionPort  ActionPortLabel=case [ 138 ]:
  Out1 : Outport
  wires:
  In1/1 -> Out1/1

== system Vehicle_Control_CodeGen/Function-Call Subsystem/If Action Subsystem8 ==
  In1 : Inport
  Action Port : ActionPort  ActionPortLabel=case [ 95 ]:
  Out1 : Outport
  wires:
  In1/1 -> Out1/1

== system Vehicle_Control_CodeGen/Function-Call Subsystem/If Action Subsystem9 ==
  In1 : Inport
  Action Port : ActionPort  ActionPortLabel=case [ 73 ]:
  Out1 : Outport
  wires:
  In1/1 -> Out1/1

== system Vehicle_Control_CodeGen/Function-Call Subsystem1/Subsystem ==
  Constant2 : Constant
  Out1 : Outport
  wires:
  Constant2/1 -> Out1/1

== system Vehicle_Control_CodeGen/Power Forcasting/Variant Subsystem ==
  note: 1) Add Subsystem or Model blocks as valid variant choices.
      | 2) You cannot connect blocks at this level. At simulation, connectivity is automatically
      | determined, based on the active variant and port name matching.
  CAN SOC : Inport
  Available Power : Inport  Port=2
  CAN Forwarding : Subsystem  VariantControl=(codegen)
  PowerUsage Simulation : Subsystem  VariantControl=(sim)
  Out1 : Outport

== system Vehicle_Control_CodeGen/Power Forcasting/Variant Subsystem1 ==
  note: 1) Add Subsystem or Model blocks as valid variant choices.
      | 2) You cannot connect blocks at this level. At simulation, connectivity is automatically
      | determined, based on the active variant and port name matching.
  In1 : Inport
  In2 : Inport  Port=2
  "Code Gen, Wheel speed averaging and integration" : Subsystem  VariantControl=(codegen)
  Fake wheel speed from simulation : Subsystem  VariantControl=(sim)
  1 : Outport

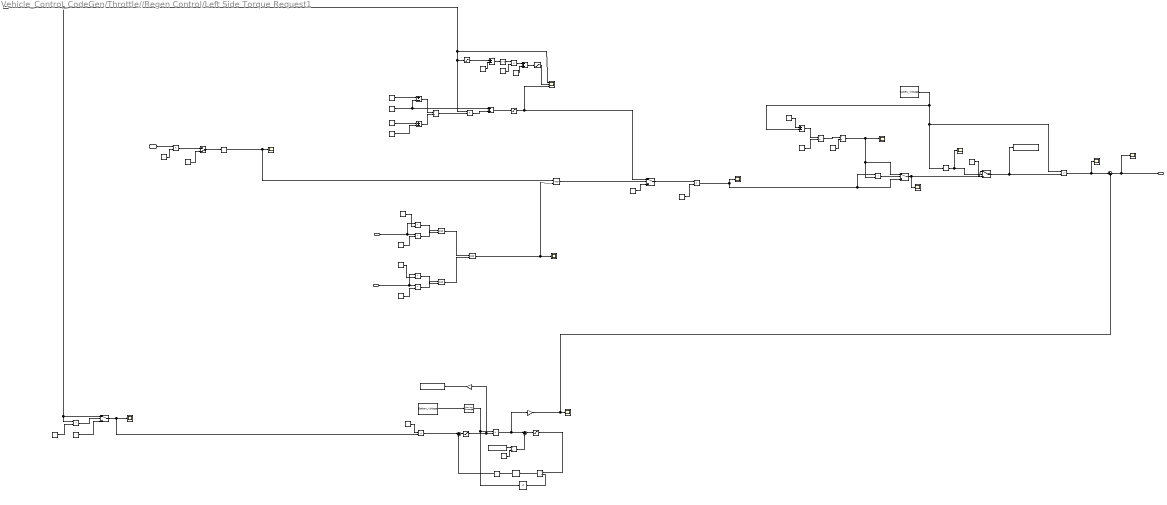
== system Vehicle_Control_CodeGen/Throttle//Regen Control/Left Side Torque Request1 ==
  note: Divide by two as the global power is the power limit for the whole vehicle, then need the left and right side power limits
  note: Halveing as this is the permissable for left/right side inverter
  note: If Conditions are not fulfilled charge current is set to zero
  note: This function was made in Desmos. Adjusted to meet cross over and start of rise
  note: Throttle pedal to regen percentage request
  note: Power Limiting to maintatin Power Limit of Less then 80 Kw
  note: Inverting as this is a discharge current
  note: throttle output enabled when less then 20% actuation, this will be used for regen
  note: If Battery Voltage greater then 590 Charge Current is set to zero
  note: Throttle Mapping to Regen Percentage
  note: Limiting the input range
  note: Speed Threshold, Regen enabled above 5km/h
  note: Max Charge Current, Regen is scalled 0-100%. Current wants to be 0 -130 amps, therfore scale by 1.3. 600V*130amps = 70kw, Then divide by two for left and right motor Control
  note: Hysterisies Control
  note: Inverting as this is a discharge current
  note: Battery Checks
  note: This is the threshold for when drive torque is requested, Regen is requested for less then 20%, and throttle is applied for greater then 22%, This gives a 2% deadband
  note: If Requested Charge current is greater then permissable charge current then switch to permisable
  In1 : Inport
  Wheel Speed (m/s) : Inport  Port=2
  Battery Temp : Inport  Port=3
  Battery SOC : Inport  Port=4
  AND{,1..3} (4 alike) : Logic  IconShape=distinctive  AllPortsSameDT=off  OutDataTypeStr=boolean
  Add2 : Sum
  Add3 : Sum
  Compare To Constant : simulink/Logic and Bit Operations/Compare To Constant  relop=>  const=5  OutDataTypeStr=boolean
  Constant : Constant  Value=2
  Constant{7,10..11,21,28} (5 alike) : Constant  Value=0
  Constant12 : Constant  Value=6
  Constant15 : Constant  Value=0.01
  Constant16 : Constant  Value=50
  Constant17 : Constant  Value=10
  Constant18 : Constant  Value=90
  Constant19 : Constant  Value=5
  Constant2 : Constant  Value=3.6
  Constant20 : Constant  Value=580
  Constant23 : Constant  Value=0.75
  Constant26 : Constant  Value=2
  Constant27 : Constant  Value=22
  Constant3 : Constant  Value=20
  Constant4 : Constant  Value=10
  Constant5 : Constant  Value=100
  Constant6 : Constant  Value=20
  Constant9 : Constant  Value=0.25
  Data Store Read : DataStoreRead  DataStoreName=Battery_Voltage  IndexOptions=Index vector (dialog)  Indices=1  OutputSizes=1
  Data Store Read1 : DataStoreRead  DataStoreName=Battery_Voltage  IndexOptions=Index vector (dialog)  Indices=1  OutputSizes=1
  Data Store Read2 : DataStoreRead  DataStoreName=Global_Power_Limit  IndexOptions=Index vector (dialog)  Indices=1  OutputSizes=1
  Data Store Write : DataStoreWrite  DataStoreName=Left_Sim_Regen_Current  IndexOptions=Index vector (dialog)  Indices=1  OutputSizes=1
  Data Store Write1 : DataStoreWrite  DataStoreName=Left_Sim_Discharge_Current  IndexOptions=Index vector (dialog)  Indices=1  OutputSizes=1
  Discrete PID Controller1 : slpidlib/PID Controller  Controller=PID  Form=Parallel  TimeDomain=Discrete-time  UseExternalTs=off  SampleTime=-1  IntegratorMethod=Forward Euler  FilterMethod=Forward Euler  ControllerParametersSource=internal  P=0.000544217300579932  I=0.544217300579932  UseKiTs=on  D=0  UseExternalDerivativeSource=off  N=100  UseFilter=on  TunerSelectOption=Transfer Function Based (PID Tuner App)  InitialConditionSource=internal  InitialConditionForIntegrator=10  InitialConditionForFilter=0  DifferentiatorICPrevScaledInput=0  ExternalReset=none  TrackingMode=off  Kt=1  LimitOutput=off  SatLimitsSource=internal  UpperSaturationLimit=inf  LowerSaturationLimit=-inf  LinearizeAsGain=off  AntiWindupMode=none  Kb=1  LimitIntegrator=off  UpperIntegratorSaturationLimit=inf  LowerIntegratorSaturationLimit=-inf  POutMin=[]  POutMax=[]  IOutMin=[]  IOutMax=[]  DOutMin=[]  DOutMax=[]  NOutMin=[]  NOutMax=[]  SumOutMin=[]  SumOutMax=[]  SaturationOutMin=[]  SaturationOutMax=[]  PParamMin=[]  PParamMax=[]  IParamMin=[]  IParamMax=[]  DParamMin=[]  DParamMax=[]  NParamMin=[]  NParamMax=[]  KbParamMin=[]  KbParamMax=[]  KtParamMin=[]  KtParamMax=[]  KbOutMin=[]  KbOutMax=[]  KtOutMin=[]  KtOutMax=[]  IntegratorOutMin=[]  IntegratorOutMax=[]  FilterOutMin=[]  FilterOutMax=[]  SumI1OutMin=[]  SumI1OutMax=[]  SumI2OutMin=[]  SumI2OutMax=[]  SumI3OutMin=[]  SumI3OutMax=[]  SumI4OutMin=[]  SumI4OutMax=[]  SumDOutMin=[]  SumDOutMax=[]  DifferentiatorOutMin=[]  DifferentiatorOutMax=[]  FilterDiffOutCoefMin=[]  FilterDiffOutCoefMax=[]  ReciprocalOutMin=[]  ReciprocalOutMax=[]  SumDenOutMin=[]  SumDenOutMax=[]  SumNumOutMin=[]  SumNumOutMax=[]  DivideOutMin=[]  DivideOutMax=[]  UdiffTsProdOutMin=[]  UdiffTsProdOutMax=[]  NTsProdOutMin=[]  NTsProdOutMax=[]  UintegralTsProdOutMin=[]  UintegralTsProdOutMax=[]  UngainTsProdOutMin=[]  UngainTsProdOutMax=[]  ClampingZeroOutDataTypeStr=Inherit: Inherit via back propagation  ClampingZeroOutMin=[]  ClampingZeroOutMax=[]  FilterDenConstantOutDataTypeStr=Inherit: Inherit via back propagation  FilterDenConstantOutMin=[]  FilterDenConstantOutMax=[]  PCopyOutDataTypeStr=Inherit: Inherit via back propagation  PCopyOutMin=[]  PCopyOutMax=[]  NCopyOutDataTypeStr=Inherit: Inherit via back propagation  NCopyOutMin=[]  NCopyOutMax=[]  IntegratorContinuousStateAttributes=''  IntegratorStateMustResolveToSignalObject=off  IntegratorRTWStateStorageClass=Auto  FilterContinuousStateAttributes=''  FilterStateMustResolveToSignalObject=off  FilterRTWStateStorageClass=Auto  ParallelPVariant=InternalParameters  IdealPVariant=Disabled  IVariant=InternalParameters  DVariant=InternalParameters  IntegratorVariant=Discrete  SatVariant=Disabled  AWVariant=Passthrough  PCopyVariant=Disabled  TRVariant=Disabled  FdbkBlocksVariant=Forward  IdealPFdbkVariant=Disabled  SatFdbkVariant=Disabled  DerivativeFilterVariant=ForwardEulerFilter  NVariant=InternalParameters  NCopyVariant=Disabled  FilterICVariant=InternalICsFilter  IntegratorICVariant=InternalICs  ExternalResetVariant=Disabled  TRSumVariant=Passthrough  SumFdbkVariant=Disabled  SumVariant=Sum_PID  TsampFilterVariant=InternalTs  TsampNgainVariant=Passthrough  TsampIntegralVariant=Disabled_SignalSpec  ExternalSaturationOutDataTypeStr=Inherit: Same as second input  DerivativeSourceVariant=ErrorSignal
      settings: LibrarySourceBlock=simulink/Discrete/Discrete PID Controller
  Divide{,1..4} (5 alike) : Product  Inputs=*/
  Gain : Gain  Gain=-1
  Gain1 : Gain  Gain=-1
  GreaterThan{,1..3} (4 alike) : RelationalOperator  Operator=>  OutDataTypeStr=boolean  RndMeth=Simplest  InputSameDT=off
  IC1 : InitialCondition  Value=600
  Less Than : RelationalOperator  Operator=<  OutDataTypeStr=boolean  RndMeth=Simplest  InputSameDT=off
  Less Than1 : RelationalOperator  Operator=<  OutDataTypeStr=boolean  RndMeth=Simplest  InputSameDT=off
  Manual Switch1 : ManualSwitch  CurrentSetting=0
  Memory1 : Memory  InitialCondition=14  InheritSampleTime=on
  Minus : Sum  Inputs=+-
  Moving Average : dspstat3/Moving Average  Method=Sliding window  ForgettingFactorPort=off  SpecifyWindowLength=on  WindowLength=10  OverlapLength=9  AllowArbitraryInputLength=off  ForgettingFactor=0.9  SimulateUsing=Interpreted execution
  Product{1..7} (7 alike) : Product
  Relay : Relay  OnSwitchValue=590  OffSwitchValue=585  OnOutputValue=0  OffOutputValue=1
  Saturation : Saturate  UpperLimit=100  LowerLimit=0
  Saturation1 : Saturate  UpperLimit=100  LowerLimit=0
  Saturation2 : Saturate  UpperLimit=20  LowerLimit=0
  Saturation3 : Saturate  UpperLimit=inf  LowerLimit=0
  Saturation5 : Saturate  UpperLimit=inf  LowerLimit=0
  Scale : Constant  Value=0.65
  Scope{,1,3,5,7..9,11,13..14} (10 alike) : Scope
  Scope2 : Scope  NumInputPorts=3
  Square : Math  Operator=square
  Subtract : Sum  Inputs=+-
  Subtract1 : Sum  Inputs=+-
  Subtract2 : Sum  Inputs=+-
  Sum : Sum  Inputs=|+-
  Sum1 : Sum  Inputs=|+-
  Sum3 : Sum  Inputs=|++
  Switch : Switch  Criteria=u2 > Threshold  SaturateOnIntegerOverflow=off  InputSameDT=off
  Switch1 : Switch  Criteria=u2 > Threshold  SaturateOnIntegerOverflow=off  InputSameDT=off
  Switch2 : Switch  Criteria=u2 > Threshold  Threshold=0.5  SaturateOnIntegerOverflow=off  InputSameDT=off
  Switch3 : Switch  Criteria=u2 > Threshold  SaturateOnIntegerOverflow=off  InputSameDT=off
  Out1 : Outport
  wires:
  Constant26/1 -> Divide4/2
  Product3/1 -> Add2/1
  Constant10/1 -> Add2/2
  Constant3/1 -> Subtract2/2
  AND/1 -> Switch/2
  Add3/1 -> Saturation/1  "Regen Request"
  GreaterThan2/1 -> Switch1/2
  Constant12/1 -> Manual Switch1/2
  GreaterThan1/1 -> AND2/1
  Constant21/1 -> Switch2/3
  In1/1 -> Switch3/1, GreaterThan3/1, Product2/1, Saturation2/1, Scope2/1  "Throttle Pedal"
  Constant11/1 -> Switch/3
  Switch3/1 -> Product6/2, Scope14/1  "Throttle Percentage > 20"
  Product5/1 -> Sum1/1, Gain1/1  "Requested Discharge Power"
  Saturation/1 -> Switch/1, Scope2/3  "Linear Regen Map"
  Switch/1 -> Product4/1  "Requested Charge Current"
  Saturation1/1 -> Scope2/2  "Exponential Throttle Map"
  Gain1/1 -> Sum3/2, Scope5/1
  Constant27/1 -> GreaterThan3/2
  Constant20/1 -> Minus/1  "Max Battery Voltage using Regen"
  Constant5/1 -> Subtract/2, Add3/1  "Max Regen Percentage"
  Constant19/1 -> GreaterThan1/2  "Min Battery SOC"
  Subtract2/1 -> Square/1
  Product7/1 -> Scope13/1, Sum3/1  "Requested Charge Power"
  Subtract/1 -> Divide1/1
  Battery SOC/1 -> GreaterThan1/1, Less Than1/1  "Battery State of Charge"
  Moving Average/1 -> IC1/1, Product5/1
  Saturation3/1 -> Divide2/1  "Power Error"
  Manual Switch1/1 -> Compare To Constant/1
  Product1/1 -> Manual Switch1/1  "Speed (km/h)"
  Subtract1/1 -> Divide1/2
  Constant17/1 -> GreaterThan/2  "Min Battery Temp"
  Saturation5/1 -> Gain/1, Product5/2
  Divide3/1 -> Sum1/2
  Product6/1 -> Sum/1  "Current Request (0-75amps)"
  Constant28/1 -> Switch3/3
  Square/1 -> Product3/1
  Saturation2/1 -> Subtract2/1  "Exponential Throttle Map"
  Sum3/1 -> Out1/1, Scope11/1
  Constant16/1 -> Less Than/2  "Max Battery temp"
  GreaterThan3/1 -> Switch3/2
  Constant6/1 -> Subtract1/1  "Minimum Throttle Percentage"
  Constant9/1 -> Product3/2
  Add2/1 -> Saturation1/1
  Wheel Speed (m/s)/1 -> Product1/1  "Speed (m/s)"
  AND3/1 -> Scope3/1, AND/2  "Battery Logic"
  Divide/1 -> Divide4/1
  Compare To Constant/1 -> AND/1, Scope1/1
  Sum/1 -> Saturation5/1
  Constant18/1 -> Less Than1/2  "Max Battery SOC"
  Constant7/1 -> Subtract1/2  "Intial distance"
  AND2/1 -> AND3/2
  Memory1/1 -> Sum/2
  AND1/1 -> AND3/1
  Constant2/1 -> Product1/2
  Data Store Read1/1 -> Minus/2, Product7/1, Relay/1
  Constant4/1 -> Subtract/1  "Min Regen Percentage"
  Less Than1/1 -> AND2/2
  Minus/1 -> Divide/1  "Voltage Threshold to overcharge"
  GreaterThan/1 -> AND1/1
  Scale/1 -> Product4/2
  Sum1/1 -> Saturation3/1
  Divide1/1 -> Product2/2  "Slope"
  Constant15/1 -> Divide/2  "Battery Internal Resistance"
  Switch2/1 -> Data Store Write/1, Product7/2  "Charge Current"
  Product4/1 -> Scope/1, Switch1/3, GreaterThan2/1  "Requested Charge Current"
  Product2/1 -> Add3/2
  Relay/1 -> Switch2/2, Scope7/1
  Battery Temp/1 -> GreaterThan/1, Less Than/1  "Battery Temp"
  Switch1/1 -> Switch2/1, Scope8/1
  Less Than/1 -> AND1/2
  Gain/1 -> Data Store Write1/1
  Divide4/1 -> GreaterThan2/2, Switch1/1, Scope9/1  "Maximum Permissable Charge Current"
  Constant23/1 -> Product6/1
  IC1/1 -> Divide2/2
  Data Store Read2/1 -> Divide3/1
  Constant/1 -> Divide3/2
  Data Store Read/1 -> Moving Average/1
  Discrete PID Controller1/1 -> Memory1/1
  Divide2/1 -> Discrete PID Controller1/1  "Current Error"

== system Vehicle_Control_CodeGen/Throttle//Regen Control/Right Side Torque Request ==
  note: Torque Request
  note: Throttle Input (%)
  note: Throttle Deadband
  note: Regen Controller
  note: Power Limit Controller (Forwards)
  note: This is the threshold for when drive torque is requested, Regen is requested for less then 20%, and throttle is applied for greater then 22%, This gives a 2% deadband
  In1 : Inport
  Wheel Speed (m/s) : Inport  Port=2
  Battery Temp : Inport  Port=3
  Battery SOC : Inport  Port=4
  Constant27 : Constant  Value=22
  Constant28 : Constant  Value=0
  GreaterThan3 : RelationalOperator  Operator=>  OutDataTypeStr=boolean  RndMeth=Simplest  InputSameDT=off
  Scope11 : Scope
  Scope13 : Scope  NumInputPorts=2
  Scope14 : Scope
  Subsystem : Subsystem
  Subsystem1 : Subsystem
  Sum3 : Sum  Inputs=|++
  Switch3 : Switch  Criteria=u2 > Threshold  SaturateOnIntegerOverflow=off  InputSameDT=off
  Out1 : Outport
  wires:
  In1/1 -> Switch3/1, GreaterThan3/1, Subsystem/1(Throttle Pedal)  "Throttle Pedal"
  Switch3/1 -> Subsystem1/1(Throttle Percentage > 20), Scope14/1  "Throttle Percentage > 20"
  Constant27/1 -> GreaterThan3/2
  Constant28/1 -> Switch3/3
  Sum3/1 -> Out1/1, Scope11/1
  GreaterThan3/1 -> Switch3/2
  Subsystem/1(Requested Charge Power) -> Scope13/1, Sum3/1
  Wheel Speed (m/s)/1 -> Subsystem/2(Speed (m/s))  "Speed (m/s)"
  Battery Temp/1 -> Subsystem/3(Battery Temp)  "Battery Temp"
  Battery SOC/1 -> Subsystem/4(Battery State of Charge)  "Battery State of Charge"
  Subsystem1/1(Out1) -> Scope13/2, Sum3/2
